simulink model "TemperaturayResistencia"  (R2022b)
settings: Solver=VariableStepAuto  StartTime=0.0  StopTime=5  RelTol=1e-3
values from neighbouring files (symbols this model uses):
  MasaBobina = 1.03    [Calculoresisytemp.m]
  Potencia = ResistenciaInicial*2*(Intensidad)^2    (= 1609.2)    [Calculoresisytemp.m]
  ResistenciaInicial = 0.894    [Calculoresisytemp.m]
  TemperaturaEntrada = 40    [Calculoresisytemp.m]
settings Model: Creator=ramuj  LastModifiedBy=ramuj

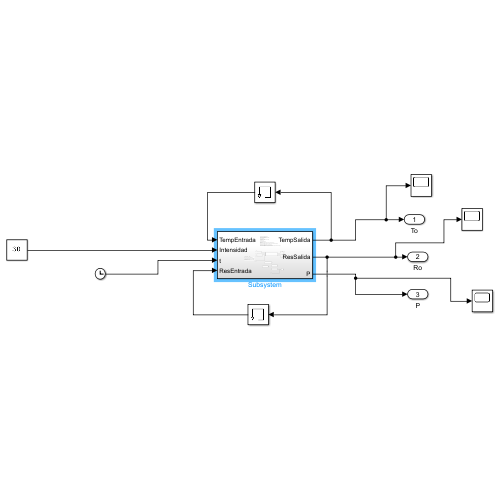
[thumbnail: Simulink's stored preview of the top-level diagram]
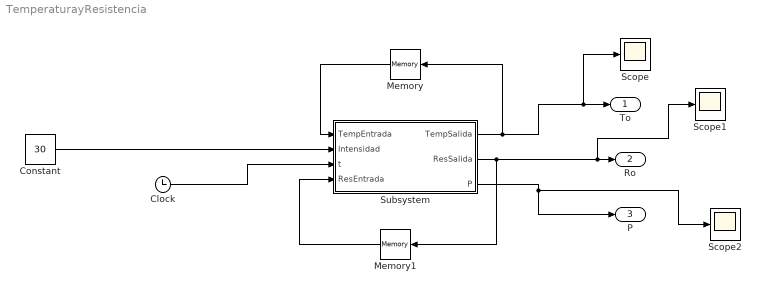
== system TemperaturayResistencia ==
  Clock : Clock
      settings: Decimation=60
  Constant : Constant  Value=30
  Memory : Memory
  Memory1 : Memory
  Scope : Scope
  Scope1 : Scope
  Scope2 : Scope
  Subsystem : Subsystem
  To : Outport
  Ro : Outport  Port=2
  P : Outport  Port=3
  wires:
  Subsystem/1(TempSalida) -> Memory/1, Scope/1, To/1
  Clock/1 -> Subsystem/3(t)
  Constant/1 -> Subsystem/2(Intensidad)
  Subsystem/2(ResSalida) -> Memory1/1, Scope1/1, Ro/1
  Subsystem/3(P) -> Scope2/1, P/1
  Memory/1 -> Subsystem/1(TempEntrada)
  Memory1/1 -> Subsystem/4(ResEntrada)

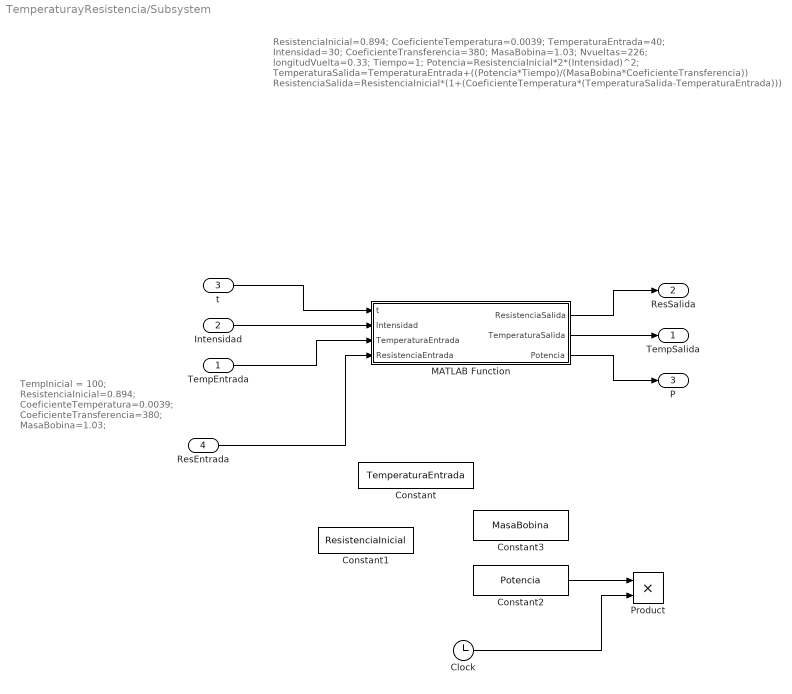
== system TemperaturayResistencia/Subsystem ==
  note: TempInicial = 100;
      | ResistenciaInicial=0.894;
      | CoeficienteTemperatura=0.0039;
      | CoeficienteTransferencia=380;
      | MasaBobina=1.03;
  note: ResistenciaInicial=0.894;
      | CoeficienteTemperatura=0.0039;
      | TemperaturaEntrada=40;
      | Intensidad=30;
      | CoeficienteTransferencia=380;
      | MasaBobina=1.03;
      | Nvueltas=226;
      | longitudVuelta=0.33;
      | Tiempo=1;
      | Potencia=ResistenciaInicial*2*(Intensidad)^2;
      | TemperaturaSalida=TemperaturaEntrada+((Potencia*Tiempo)/(MasaBobina*CoeficienteTransferencia))
      | ResistenciaSalida=ResistenciaInicial*(1+(CoeficienteTemperatura*(TemperaturaSalida-TemperaturaEntrada)))
  TempEntrada : Inport
  Intensidad : Inport  Port=2
  t : Inport  Port=3
  ResEntrada : Inport  Port=4
  Clock : Clock
  Constant : Constant  Value=TemperaturaEntrada
  Constant1 : Constant  Value=ResistenciaInicial
  Constant2 : Constant  Value=Potencia
  Constant3 : Constant  Value=MasaBobina
  MATLAB Function : MATLAB Function  TreatAsAtomicUnit=on
  Product : Product
  TempSalida : Outport
  ResSalida : Outport  Port=2
  P : Outport  Port=3
  wires:
  Intensidad/1 -> MATLAB Function/2(Intensidad)
  t/1 -> MATLAB Function/1(t)
  MATLAB Function/1(ResistenciaSalida) -> ResSalida/1
  MATLAB Function/2(TemperaturaSalida) -> TempSalida/1
  MATLAB Function/3(Potencia) -> P/1
  ResEntrada/1 -> MATLAB Function/4(ResistenciaEntrada)
  TempEntrada/1 -> MATLAB Function/3(TemperaturaEntrada)
  Constant2/1 -> Product/1
  Clock/1 -> Product/2

== matlab function TemperaturayResistencia/Subsystem/MATLAB Function ==
  data: t input; Intensidad input; ResistenciaSalida output; TemperaturaSalida output; Potencia output; TemperaturaEntrada input; ResistenciaEntrada input
function [ResistenciaSalida, TemperaturaSalida, Potencia] = fcn(t, Intensidad, TemperaturaEntrada, ResistenciaEntrada)

TempInicial = 100;
ResistenciaInicial=0.894;
CoeficienteTemperatura=0.0039;
CoeficienteTransferencia=380;
MasaBobina=1.03;
%Nvueltas=226;
%longitudVuelta=0.33;

if(t == 0)
    TemperaturaSalida = TempInicial;
    ResistenciaSalida=ResistenciaInicial;
    Potencia=ResistenciaInicial*2*(Intensidad)^2;
else

    t2 = t;
    aux = t2;
    t1 = aux;
    Tiempo = 1;

    Potencia=ResistenciaEntrada*2*(Intensidad)^2;
    TemperaturaSalida=TemperaturaEntrada+((Potencia*Tiempo)/(MasaBobina*CoeficienteTransferencia));
    ResistenciaSalida=ResistenciaEntrada*(1+(CoeficienteTemperatura*(TemperaturaSalida-TemperaturaEntrada)));

end
